simulink model "AR_Drone_Flight_Control"  (R2014a)
settings: configuration reference "AR_Drone_ConfigSet" (kept outside this file)
values from neighbouring files (symbols this model uses):
  Accelerometer_quick_calibration = [0.003485 0.008674 -0.9985]    [Calibration_Parameters.mat]
  Gyrometer_quick_calibration = [-10.63 2.778 -0.1868]    [Calibration_Parameters.mat]
undefined symbols (not defined in the file or in its folder): Accelerometer_360deg_calibration, Drone_StateModeType, Magnetometer_calibration, Navigation, Navigation_KF_Lib, sigbuilder_block
libraries: simulink x15, vrlib x7, aerolibtransform2 x5, AR_Drone_2_Library x4, dspnetwork x3, aerolibutil x2
(part 1 of 3)
settings Model: SimulationMode=external  ExtModeTrigDuration=48000  Creator=nraman  LastModifiedBy=Raphaël

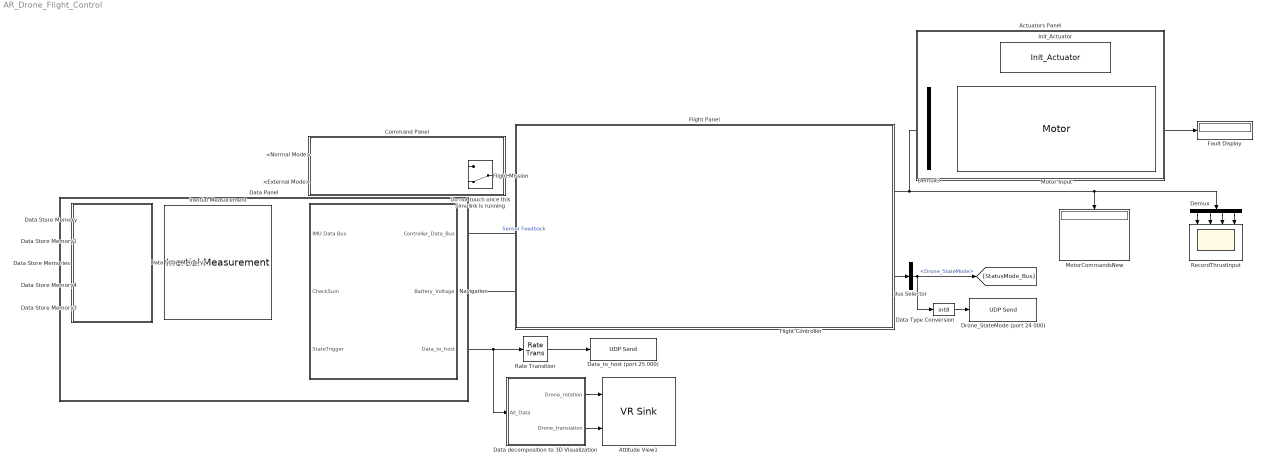
== system AR_Drone_Flight_Control ==
  <External Mode> : Subsystem
  <Normal Mode> : Subsystem
  Actuators Panel : Subsystem
  Attitude View1 : vrlib/VR Sink  InstantiateOnLoad=on  SampleTime=-1  ViewEnable=on  RemoteChange=off  RemoteView=off  FieldsWritten=Drone.rotation.4.1.1.double#Drone.translation.3.1.1.double  WorldFileName=myDrone3.wrl  AutoView=off  VideoDimensions=[]  AllowVariableSize=off
  Bus Selector : BusSelector  OutputSignals=Drone_StateMode
  Command Panel : Subsystem
  Data Panel : Subsystem
  Data Store Memory : DataStoreMemory  DataStoreName=Offset_Accel  ReadBeforeWriteMsg=warning  WriteAfterWriteMsg=warning  WriteAfterReadMsg=warning  InitialValue=[0 0 0]  OutDataTypeStr=double
  Data Store Memory1 : DataStoreMemory  DataStoreName=Offset_Gyro  ReadBeforeWriteMsg=warning  WriteAfterWriteMsg=warning  WriteAfterReadMsg=warning  InitialValue=[0 0 0]  OutDataTypeStr=double
  Data Store Memory2 : DataStoreMemory  DataStoreName=Input_ports  ReadBeforeWriteMsg=warning  WriteAfterWriteMsg=warning  WriteAfterReadMsg=warning  InitialValue=[0 0]  OutDataTypeStr=double
  Data Store Memory3 : DataStoreMemory  DataStoreName=Output_ports  ReadBeforeWriteMsg=warning  WriteAfterWriteMsg=warning  WriteAfterReadMsg=warning  InitialValue=[0 0]  OutDataTypeStr=double
  Data Store Memory4 : DataStoreMemory  DataStoreName=Flight_Mission_On_Off  ReadBeforeWriteMsg=warning  WriteAfterWriteMsg=warning  WriteAfterReadMsg=warning  InitialValue=false  OutDataTypeStr=boolean
  Data Store Memories : Subsystem
  Data Type Conversion : DataTypeConversion  OutDataTypeStr=int8
  Data decomposition to 3D Visualization : Subsystem
  Data_to_host (port 25 000) : dspnetwork/UDP Send  remoteURL=Host_IP_Adress  remotePort=25000  localURL='0.0.0.0'  localPortSource=Automatically determine  localPort=-1  sampletime=-1  blockPlatform=LINUX  separateLengthPort=0
  Demux : Demux
  Demux3 : Demux
  Do not touch once this Simulink is running : ManualSwitch  CurrentSetting=0
  Drone_StateMode (port 24 000) : dspnetwork/UDP Send  remoteURL=Host_IP_Adress  remotePort=24000  localURL='0.0.0.0'  localPortSource=Automatically determine  localPort=-1  sampletime=-1  blockPlatform=LINUX  separateLengthPort=0
  Fault Display : Display
  Flight Controller : Subsystem
  Flight Mission : Subsystem
  Flight Panel : Subsystem
  Inertial Measurement : AR_Drone_2_Library/Inertial Measurement  Ts=1/400
  Init_Actuator : AR_Drone_2_Library/Init_Actuator  ShowSpec=on
  Motor Input : AR_Drone_2_Library/Motor
  MotorCommandsNew : Display
  Navigation : Subsystem  AncestorBlock=Navigation_KF_Lib/Navigation
      mask DialogControl DescTextVar Prompt: Kalman Filter Navigation Implementation
  Rate Transition : RateTransition  OutPortSampleTime=2/400
  RecordThrustInput : Scope  NumInputPorts=4
      settings: TimeRange=44.32823813354787  YMin=20~20~-5~-5  YMax=85~90~5~5  SaveName=Control_Input
  wires:
  Motor Input/1 -> Fault Display/1
  Demux3/1 -> Motor Input/1
  Demux3/2 -> Motor Input/2
  Demux3/3 -> Motor Input/3
  Demux3/4 -> Motor Input/4
  Inertial Measurement/1 -> Navigation/1(IMU Data Bus)
  Inertial Measurement/2 -> Navigation/2(CheckSum)
  Flight Controller/2(ControlStatus_Bus) -> Bus Selector/1
  Demux/1 -> RecordThrustInput/1
  Demux/2 -> RecordThrustInput/2
  Navigation/1(Controller_Data_Bus) -> Flight Controller/2(Controller Feedback Data Bus)  "Sensor Feedback"
  Navigation/2(Battery_Voltage) -> Flight Controller/3(BatteryVoltage)
  [StatusMode_Bus] -> Navigation/3(StateTrigger)
  Navigation/3(Data_to_host) -> Rate Transition/1, Data decomposition to 3D Visualization/1(All_Data)
  Data decomposition to 3D Visualization/1(Drone_rotation) -> Attitude View1/1
  Data decomposition to 3D Visualization/2(Drone_translation) -> Attitude View1/2
  Flight Controller/1(MotorCommand) -> Demux3/1, MotorCommandsNew/1, Demux/1
  Demux/3 -> RecordThrustInput/3
  Demux/4 -> RecordThrustInput/4
  Bus Selector/1 -> [StatusMode_Bus], Data Type Conversion/1  "<Drone_StateMode>"
  Data Type Conversion/1 -> Drone_StateMode (port 24 000)/1
  Rate Transition/1 -> Data_to_host (port 25 000)/1
  Flight Mission/1(Command) -> Flight Controller/1(Command)
  <External Mode>/1("<External Mode> (on PC) : Switch") -> Do not touch once this Simulink is running/2
  Do not touch once this Simulink is running/1 -> Flight Mission/1(Start/Stop)
  <Normal Mode>/1("<Normal Mode> (Embedded) : UDP") -> Do not touch once this Simulink is running/1

== system AR_Drone_Flight_Control/<External Mode> ==
  " 1" : DataTypeConversion  OutDataTypeStr=int16
  Constant2 : Constant  Value=+1
  Constant3 : Constant  Value=-1
  Switch to change the current Drone State (it has to be down at the start) : ManualSwitch  CurrentSetting=0
  "<External Mode> (on PC) : Switch" : Outport
  wires:
  " 1"/1 -> "<External Mode> (on PC) : Switch"/1
  Switch to change the current Drone State (it has to be down at the start)/1 -> " 1"/1
  Constant2/1 -> Switch to change the current Drone State (it has to be down at the start)/1
  Constant3/1 -> Switch to change the current Drone State (it has to be down at the start)/2

== system AR_Drone_Flight_Control/<Normal Mode> ==
  " 1" : DataTypeConversion  OutDataTypeStr=int16
  Host Command (port 7 000) : dspnetwork/UDP Receive  localURL='0.0.0.0'  localPort=6000  remoteURL='0.0.0.0'  remotePort=-1  recvBufferSize=8192  dims=1  signalDatatype=double  isVarSize=off  showBlockingTime=on  blockingTime=0  sampletime=1/400  blockPlatform=LINUX
  Terminator2 : Terminator
  "<Normal Mode> (Embedded) : UDP" : Outport
  wires:
  Host Command (port 7 000)/2 -> Terminator2/1
  Host Command (port 7 000)/1 -> " 1"/1
  " 1"/1 -> "<Normal Mode> (Embedded) : UDP"/1

== system AR_Drone_Flight_Control/Actuators Panel ==

== system AR_Drone_Flight_Control/Command Panel ==

== system AR_Drone_Flight_Control/Data Panel ==

== system AR_Drone_Flight_Control/Data Store Memories ==

== system AR_Drone_Flight_Control/Data decomposition to 3D Visualization ==
  All_Data : Inport
  DCM (diagonal = 1 / else 0) : Display
      settings: Decimation=3
  Demux7 : Demux  Outputs=[13 9 3 3 3 3]
  Reshape : Reshape  OutputDimensionality=Customize  OutputDimensions=[3,3]
  SL3D Visualization1 : Subsystem
  Terminator2 : Terminator
  Terminator3 : Terminator
  Drone_rotation : Outport
  Drone_translation : Outport  Port=2
  wires:
  All_Data/1 -> Demux7/1
  Demux7/3 -> SL3D Visualization1/2(GravVector)
  Demux7/4 -> SL3D Visualization1/3(MagXY)
  Demux7/5 -> SL3D Visualization1/4(MagVector)
  Reshape/1 -> DCM (diagonal = 1 / else 0)/1, SL3D Visualization1/1(VisualizationInput)
  SL3D Visualization1/1(VRML_out) -> Drone_rotation/1
  SL3D Visualization1/2(VRML_pos) -> Drone_translation/1
  Demux7/2 -> Reshape/1
  Demux7/6 -> Terminator3/1
  Demux7/1 -> Terminator2/1

== system AR_Drone_Flight_Control/Flight Controller ==
  Command : Inport
  Controller Feedback Data Bus : Inport  Port=2
  BatteryVoltage : Inport  Port=3
  Bus Creator : BusCreator  Inputs=5
  Bus Selector : BusSelector  OutputSignals=UltraSound,EulerAngles,ProcessedGyro,AccelNorm
  Bus Selector1 : BusSelector  OutputSignals=Desired_Drone_StateMode,Auto-Calibration_ON_OFF,Altitude_ON_OFF,Desired_Roll_Pitch_Yaw
  Data Type Conversion1 : DataTypeConversion  OutDataTypeStr=int16
  Data Type Conversion3 : DataTypeConversion  OutDataTypeStr=int16
  Data Type Conversion4 : DataTypeConversion  OutDataTypeStr=int16
  Data Type Conversion5 : DataTypeConversion  OutDataTypeStr=boolean
  Drone_State-Mode Conversion : DataTypeConversion  OutDataTypeStr=Enum: Drone_StateModeType
  FilterBattVoltage : DiscreteTransferFcn  Numerator=[ 0.07226]  Denominator=[1 -0.9277]  SampleTime=1/400
  Nominal Thrust : Constant  Value=55  OutDataTypeStr=int16
  Selector : Selector  InputPortWidth=3  Indices=[3]
  Supervisory Flight Controller : Stateflow chart  TreatAsAtomicUnit=on
  MotorCommand : Outport
  ControlStatus_Bus : Outport  Port=2
  wires:
  Supervisory Flight Controller/1(MotorCmd) -> Bus Creator/1, MotorCommand/1
  Supervisory Flight Controller/2(" Drone_StateMode") -> Bus Creator/2
  Bus Selector/1 -> Supervisory Flight Controller/5(UltraSound_Feedback)  "<UltraSound>"
  Controller Feedback Data Bus/1 -> Bus Selector/1
  [Accel_data_for_offset] -> Supervisory Flight Controller/11(Accel_Measures_for_Offset)
  Supervisory Flight Controller/5(refHeight) -> Bus Creator/5
  [Gyro_data_for_offset] -> Supervisory Flight Controller/12(Gyro_Measures_for_Offset)
  BatteryVoltage/1 -> FilterBattVoltage/1
  FilterBattVoltage/1 -> Supervisory Flight Controller/10(Measured_Battery_Voltage)
  Selector/1 -> Supervisory Flight Controller/8(AccelVector_Input)
  Supervisory Flight Controller/3(" BatteryFault_Mode") -> Bus Creator/3
  Supervisory Flight Controller/4(" SafeOrientation_Mode") -> Bus Creator/4
  Bus Creator/1 -> ControlStatus_Bus/1  "StatusMode_Bus"
  Bus Selector/4 -> Selector/1  "<AccelNorm>"
  Bus Selector/2 -> Supervisory Flight Controller/6(Euler_Angles)  "<EulerAngles>"
  Bus Selector/3 -> Supervisory Flight Controller/7(Angular_Velocity)  "<ProcessedGyro>"
  Data Type Conversion1/1 -> Drone_State-Mode Conversion/1
  Drone_State-Mode Conversion/1 -> Supervisory Flight Controller/1(hostCmd)
  Data Type Conversion4/1 -> Supervisory Flight Controller/3(EnableAltitudeCtrl)
  Command/1 -> Bus Selector1/1
  Data Type Conversion5/1 -> Supervisory Flight Controller/2(Auto_Calibration)
  Nominal Thrust/1 -> Data Type Conversion3/1
  Data Type Conversion3/1 -> Supervisory Flight Controller/9(NominalThrust)
  Bus Selector1/1 -> Data Type Conversion1/1  "<Desired_Drone_StateMode>"
  Bus Selector1/4 -> Supervisory Flight Controller/4(Desired_Attitude_deg)  "<Desired_Roll_Pitch_Yaw>"
  Bus Selector1/3 -> Data Type Conversion4/1  "<Altitude_ON_OFF>"
  Bus Selector1/2 -> Data Type Conversion5/1  "<Auto-Calibration_ON_OFF>"

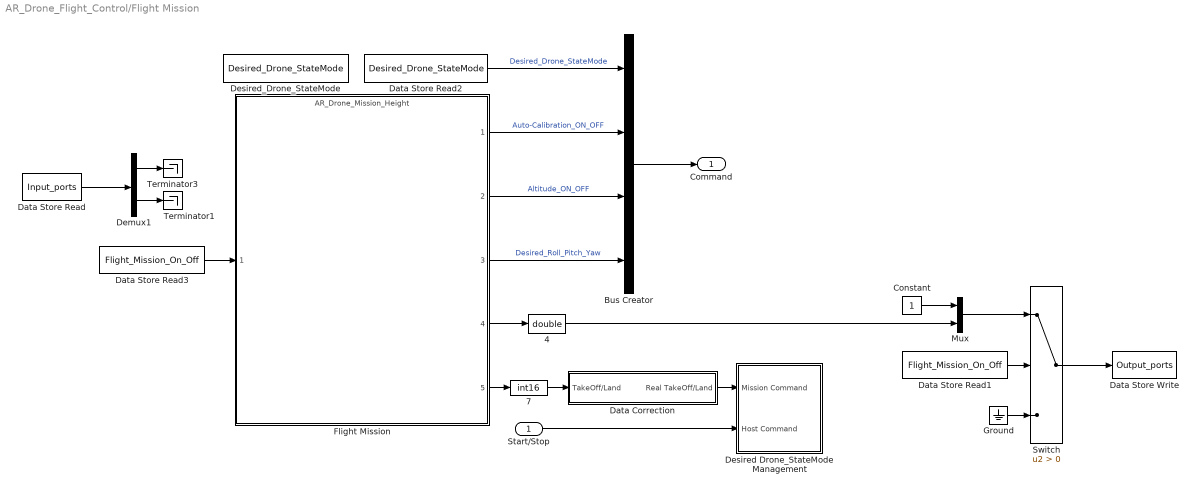
== system AR_Drone_Flight_Control/Flight Mission ==
  Start/Stop : Inport
  " 4" : DataTypeConversion  OutDataTypeStr=double
  " 7" : DataTypeConversion  OutDataTypeStr=int16
  Bus Creator : BusCreator
  Constant : Constant
  Data Correction : Subsystem
  Data Store Read : DataStoreRead  DataStoreName=Input_ports
  Data Store Read1 : DataStoreRead  DataStoreName=Flight_Mission_On_Off
  Data Store Read2 : DataStoreRead  DataStoreName=Desired_Drone_StateMode
  Data Store Read3 : DataStoreRead  DataStoreName=Flight_Mission_On_Off
  Data Store Write : DataStoreWrite  DataStoreName=Output_ports
  Demux1 : Demux  Outputs=2
  Desired Drone_StateMode Management : Subsystem
  Desired_Drone_StateMode : DataStoreMemory  DataStoreName=Desired_Drone_StateMode  ReadBeforeWriteMsg=warning  WriteAfterWriteMsg=warning  WriteAfterReadMsg=warning  InitialValue=Drone_StateModeType.Landing_Sequence  OutDataTypeStr=Enum: Drone_StateModeType
  Flight Mission : ModelReference  ModelNameDialog=AR_Drone_Mission_Height.slx  SimulationMode=Normal  ModelReferenceVersion=1.1120  CopyOfModelName=AR_Drone_Mission_Height.slx  DefaultDataLogging=on
  Ground : Ground
  Mux : Mux  Inputs=2
  Switch : Switch  Criteria=u2 > Threshold
  Terminator1 : Terminator
  Terminator3 : Terminator
  Command : Outport
  wires:
  Ground/1 -> Switch/3
  Flight Mission/5 -> " 7"/1
  Mux/1 -> Switch/1
  Constant/1 -> Mux/1
  Data Store Read3/1 -> Flight Mission/1
  Data Store Read/1 -> Demux1/1
  Demux1/2 -> Terminator1/1
  Switch/1 -> Data Store Write/1
  Flight Mission/1 -> Bus Creator/2  "Auto-Calibration_ON_OFF"
  Flight Mission/2 -> Bus Creator/3  "Altitude_ON_OFF"
  Flight Mission/3 -> Bus Creator/4  "Desired_Roll_Pitch_Yaw"
  Flight Mission/4 -> " 4"/1
  Start/Stop/1 -> Desired Drone_StateMode Management/2(Host Command)
  Data Store Read2/1 -> Bus Creator/1  "Desired_Drone_StateMode"
  " 4"/1 -> Mux/2
  " 7"/1 -> Data Correction/1(TakeOff/Land)
  Data Store Read1/1 -> Switch/2
  Data Correction/1(Real TakeOff/Land) -> Desired Drone_StateMode Management/1(Mission Command)
  Bus Creator/1 -> Command/1
  Demux1/1 -> Terminator3/1

== system AR_Drone_Flight_Control/Flight Panel ==

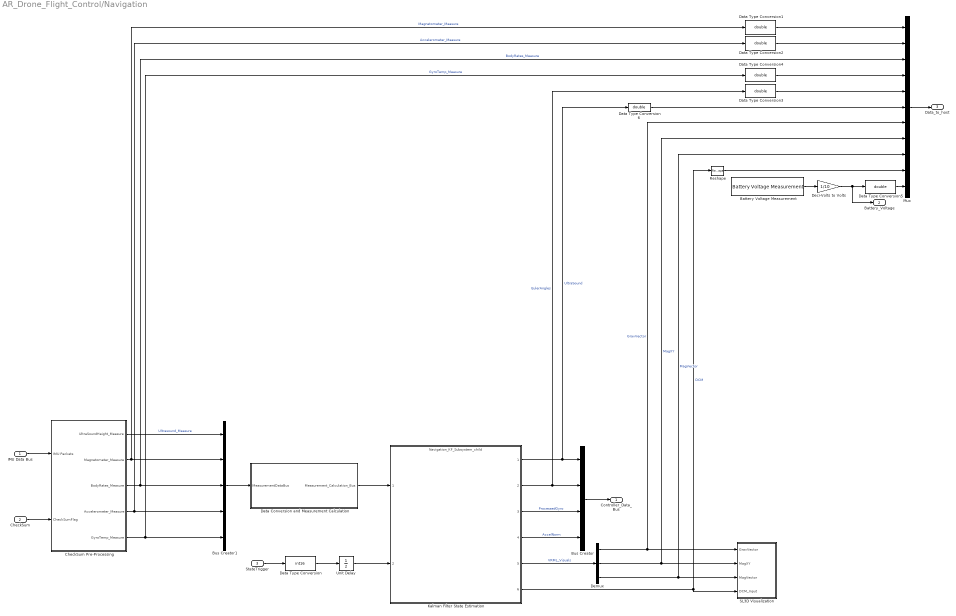
== system AR_Drone_Flight_Control/Navigation ==
  IMU Data Bus : Inport  OutDataTypeStr=Bus: IMU_Packets
  CheckSum : Inport  Port=2
  StateTrigger : Inport  Port=3  OutDataTypeStr=Enum: Drone_StateModeType
  Battery Voltage Measurement : AR_Drone_2_Library/Battery Voltage Measurement  SFunctionSpec=void BatteryMeasure_step(single y1[1])  SampleTime=1/400
  Bus Creator : BusCreator
  Bus Creator1 : BusCreator  Inputs=5
  CheckSum Pre-Processing : Subsystem  TreatAsAtomicUnit=on
      settings: RTWSystemCode=Inline
  Data Conversion and Measurement Calculation : Subsystem
  Data Type Conversion : DataTypeConversion  OutDataTypeStr=int16
  Data Type Conversion{1..6} (6 alike) : DataTypeConversion  OutDataTypeStr=double
  Deci-Volts to Volts : Gain  Gain=1/10
  Demux : Demux  Outputs=[3 3 3]
  Kalman Filter State Estimation : ModelReference  ModelNameDialog=Navigation_KF_Subsystem_child.slx  SimulationMode=Normal  ModelReferenceVersion=1.63  CopyOfModelName=Navigation_KF_Subsystem_child.slx  DefaultDataLogging=on
  Mux : Mux  Inputs=11
  Reshape : Reshape
  SL3D Visualization : Subsystem
  Unit Delay : UnitDelay  SampleTime=-1
  Controller_Data_Bus : Outport
  Battery_Voltage : Outport  Port=2
  Data_to_host : Outport  Port=3
  wires:
  Kalman Filter State Estimation/4 -> Bus Creator/4  "AccelNorm"
  Kalman Filter State Estimation/3 -> Bus Creator/3  "ProcessedGyro"
  StateTrigger/1 -> Data Type Conversion/1
  Bus Creator1/1 -> Data Conversion and Measurement Calculation/1(MeasurementDataBus)
  CheckSum Pre-Processing/5(GyroTemp_Measure) -> Data Type Conversion4/1, Bus Creator1/5  "GyroTemp_Measure"
  CheckSum Pre-Processing/4(Accelerometer_Measure) -> Data Type Conversion2/1, Bus Creator1/4  "Accelerometer_Measure"
  CheckSum Pre-Processing/3(BodyRates_Measure) -> Mux/3, Bus Creator1/3  "BodyRates_Measure"
  CheckSum Pre-Processing/2(Magnetometer_Measure) -> Data Type Conversion1/1, Bus Creator1/2  "Magnetometer_Measure"
  CheckSum Pre-Processing/1(UltraSoundHeight_Measure) -> Bus Creator1/1  "Ultrasound_Measure"
  CheckSum/1 -> CheckSum Pre-Processing/2(CheckSumFlag)
  IMU Data Bus/1 -> CheckSum Pre-Processing/1(IMU Packets)
  Unit Delay/1 -> Kalman Filter State Estimation/2
  Data Type Conversion/1 -> Unit Delay/1
  Kalman Filter State Estimation/1 -> Data Type Conversion6/1, Bus Creator/1  "UltraSound"
  Demux/1 -> Mux/7, SL3D Visualization/1(GravVector)  "GravVector"
  Demux/3 -> Mux/9, SL3D Visualization/3(MagVector)  "MagVector"
  Bus Creator/1 -> Controller_Data_Bus/1
  Kalman Filter State Estimation/2 -> Data Type Conversion3/1, Bus Creator/2  "EulerAngles"
  Kalman Filter State Estimation/5 -> Demux/1  "VRML_Visuals"
  Demux/2 -> Mux/8, SL3D Visualization/2(MagXY)  "MagXY"
  Data Conversion and Measurement Calculation/1(Measurement_Calculation_Bus) -> Kalman Filter State Estimation/1
  Kalman Filter State Estimation/6 -> SL3D Visualization/4(DCM_Input), Reshape/1  "DCM"
  Data Type Conversion4/1 -> Mux/4
  Data Type Conversion3/1 -> Mux/5
  Data Type Conversion2/1 -> Mux/2
  Data Type Conversion1/1 -> Mux/1
  Mux/1 -> Data_to_host/1
  Reshape/1 -> Mux/10
  Data Type Conversion6/1 -> Mux/6
  Battery Voltage Measurement/1 -> Deci-Volts to Volts/1
  Deci-Volts to Volts/1 -> Battery_Voltage/1, Data Type Conversion5/1
  Data Type Conversion5/1 -> Mux/11

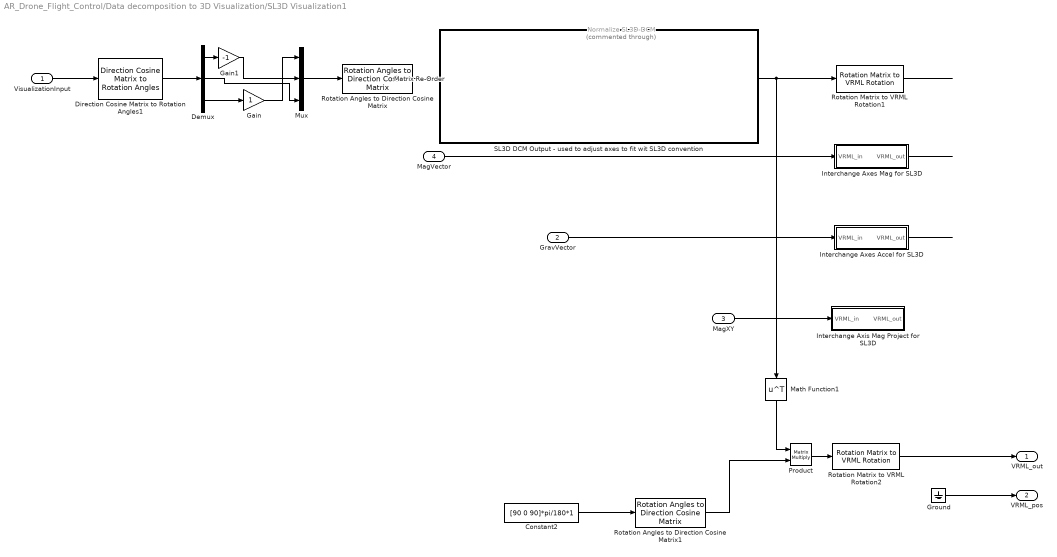
== system AR_Drone_Flight_Control/Data decomposition to 3D Visualization/SL3D Visualization1 ==
  VisualizationInput : Inport
  GravVector : Inport  Port=2
  MagXY : Inport  Port=3
  MagVector : Inport  Port=4
  Constant2 : Constant  Value=[90 0 90]*pi/180*1
  Demux : Demux  Outputs=3
  Direction Cosine Matrix to Rotation Angles1 : aerolibtransform2/Direction Cosine Matrix to Rotation Angles  rotationOrder=XYZ  lim=ZeroR3
      settings: AttributesFormatString=Rotation Order: %<rotationOrder>
  Gain : Gain  OutDataTypeStr=Inherit: Same as input
  Gain1 : Gain  Gain=-1  OutDataTypeStr=Inherit: Same as input
  Ground : Ground
  "Interchange Axes Accel for SL3D " : Subsystem
  "Interchange Axes Mag for SL3D " : Subsystem
  Interchange Axis Mag Project for SL3D : Subsystem
  Math Function1 : Math  Operator=transpose  SaturateOnIntegerOverflow=on
  Matrix Re-Order : MATLAB Function  TreatAsAtomicUnit=on
  Mux : Mux  Inputs=3
  Normalize SL3D-DCM : Subsystem  Commented=through  TreatAsAtomicUnit=on
  Product : Product  Multiplication=Matrix(*)
  Rotation Angles to Direction Cosine Matrix : aerolibtransform2/Rotation Angles to Direction Cosine Matrix  rotationOrder=XYZ
  Rotation Angles to Direction Cosine Matrix1 : aerolibtransform2/Rotation Angles to Direction Cosine Matrix  rotationOrder=XYZ
  Rotation Matrix to VRML Rotation1 : vrlib/Utilities/Rotation Matrix to VRML Rotation  maxzero=1e-12
  Rotation Matrix to VRML Rotation2 : vrlib/Utilities/Rotation Matrix to VRML Rotation  maxzero=1e-12
  SL3D DCM Output - used to adjust axes to fit wit SL3D convention : Subsystem
  VRML_out : Outport
  VRML_pos : Outport  Port=2
  wires:
  Rotation Matrix to VRML Rotation1/1 -> ?
  "Interchange Axes Accel for SL3D "/1(VRML_out) -> ?
  VisualizationInput/1 -> Direction Cosine Matrix to Rotation Angles1/1
  GravVector/1 -> "Interchange Axes Accel for SL3D "/1(VRML_in)
  Matrix Re-Order/1(M_out) -> Normalize SL3D-DCM/1(DCM)
  Direction Cosine Matrix to Rotation Angles1/1 -> Demux/1
  Demux/3 -> Gain/1
  Mux/1 -> Rotation Angles to Direction Cosine Matrix/1
  "Interchange Axes Mag for SL3D "/1(VRML_out) -> ?
  MagVector/1 -> "Interchange Axes Mag for SL3D "/1(VRML_in)
  Rotation Angles to Direction Cosine Matrix/1 -> Matrix Re-Order/1(M_in)
  MagXY/1 -> Interchange Axis Mag Project for SL3D/1(VRML_in)
  Rotation Matrix to VRML Rotation2/1 -> VRML_out/1
  Constant2/1 -> Rotation Angles to Direction Cosine Matrix1/1
  Rotation Angles to Direction Cosine Matrix1/1 -> Product/2
  Product/1 -> Rotation Matrix to VRML Rotation2/1
  Normalize SL3D-DCM/1(DCM_normalized) -> Math Function1/1, Rotation Matrix to VRML Rotation1/1
  Math Function1/1 -> Product/1
  Gain/1 -> Mux/1
  Demux/1 -> Gain1/1
  Demux/2 -> Mux/3
  Gain1/1 -> Mux/2
  Ground/1 -> VRML_pos/1

== system AR_Drone_Flight_Control/Flight Controller/Supervisory Flight Controller/Altitude_Control ==
  note: Thurst Table
      | _________________
      | At 100cm error  - 20% duty cycle - saturation : 10
      | 80 cm error - 16% duty cycle - saturation
      | 70 cm error - 14% duty cycle - saturation
      | 60 cm error - 12% duty cycle
  HeightFeedback : Inport  OutDataTypeStr=double  PortDimensions=2
  refHeight : Inport  Port=2  OutDataTypeStr=double  PortDimensions=1
  f : TriggerPort  TriggerType=function-call
      settings: CopyFcn=Stateflow.SLINSF.SimulinkMan.removeBlockPreDeleteFcn  PreDeleteFcn=Stateflow.SLINSF.SimulinkMan.unsafePredeleteFcn
  Control Effort : Scope
      settings: YMin=8.735  YMax=8.7875  SaveName=ScopeData3
  Data Type Conversion1 : DataTypeConversion  OutDataTypeStr=int16
  Demux : Demux  Outputs=2
  Discrete PID Controller _ WORKING1 : simulink/Continuous/PID Controller  Commented=on  Controller=PID  TimeDomain=Discrete-time  SampleTime=-1  IntegratorMethod=Forward Euler  FilterMethod=Forward Euler  Form=Parallel  P=0.387369235850492*0.7  I=0.018136*4  D=0.819231727791919*0.15  N=12.5907330811849  InitialConditionSource=internal  InitialConditionForIntegrator=0  InitialConditionForFilter=0  ExternalReset=none  LimitOutput=on  UpperSaturationLimit=20  LowerSaturationLimit=-20  LinearizeAsGain=off  AntiWindupMode=clamping  Kb=1  TrackingMode=off  Kt=1  PParamMin=[]  PParamMax=[]  IParamMin=[]  IParamMax=[]  DParamMin=[]  DParamMax=[]  NParamMin=[]  NParamMax=[]  KbParamMin=[]  KbParamMax=[]  KtParamMin=[]  KtParamMax=[]  POutMin=[]  POutMax=[]  IOutMin=[]  IOutMax=[]  DOutMin=[]  DOutMax=[]  NOutMin=[]  NOutMax=[]  KbOutMin=[]  KbOutMax=[]  KtOutMin=[]  KtOutMax=[]  IntegratorOutMin=[]  IntegratorOutMax=[]  FilterOutMin=[]  FilterOutMax=[]  SumOutMin=[]  SumOutMax=[]  SumI1OutMin=[]  SumI1OutMax=[]  SumI2OutMin=[]  SumI2OutMax=[]  SumI3OutMin=[]  SumI3OutMax=[]  SumDOutMin=[]  SumDOutMax=[]  SaturationOutMin=[]  SaturationOutMax=[]  IntegratorContinuousStateAttributes=''  IntegratorStateMustResolveToSignalObject=off  IntegratorRTWStateStorageClass=Auto  FilterContinuousStateAttributes=''  FilterStateMustResolveToSignalObject=off  FilterRTWStateStorageClass=Auto
  Display3 : Display
  Height Error : Scope  NumInputPorts=2
      settings: ShowLegends=on  YMin=-0.1075~-5  YMax=-0.08~5  SaveName=ScopeData13
  PID_Smooth : simulink/Continuous/PID Controller  Controller=PID  TimeDomain=Discrete-time  SampleTime=-1  IntegratorMethod=Forward Euler  FilterMethod=Forward Euler  Form=Parallel  P=0.387369235850492*0.9  I=0.018136*4  D=0.819231727791919*0.2  N=12.5907330811849  InitialConditionSource=internal  InitialConditionForIntegrator=0  InitialConditionForFilter=0  ExternalReset=none  LimitOutput=on  UpperSaturationLimit=20  LowerSaturationLimit=-20  LinearizeAsGain=off  AntiWindupMode=clamping  Kb=1  TrackingMode=off  Kt=1  PParamMin=[]  PParamMax=[]  IParamMin=[]  IParamMax=[]  DParamMin=[]  DParamMax=[]  NParamMin=[]  NParamMax=[]  KbParamMin=[]  KbParamMax=[]  KtParamMin=[]  KtParamMax=[]  POutMin=[]  POutMax=[]  IOutMin=[]  IOutMax=[]  DOutMin=[]  DOutMax=[]  NOutMin=[]  NOutMax=[]  KbOutMin=[]  KbOutMax=[]  KtOutMin=[]  KtOutMax=[]  IntegratorOutMin=[]  IntegratorOutMax=[]  FilterOutMin=[]  FilterOutMax=[]  SumOutMin=[]  SumOutMax=[]  SumI1OutMin=[]  SumI1OutMax=[]  SumI2OutMin=[]  SumI2OutMax=[]  SumI3OutMin=[]  SumI3OutMax=[]  SumDOutMin=[]  SumDOutMax=[]  SaturationOutMin=[]  SaturationOutMax=[]  IntegratorContinuousStateAttributes=''  IntegratorStateMustResolveToSignalObject=off  IntegratorRTWStateStorageClass=Auto  FilterContinuousStateAttributes=''  FilterStateMustResolveToSignalObject=off  FilterRTWStateStorageClass=Auto
  Re-Calibrate : Saturate  UpperLimit=200  LowerLimit=0  OutMin=0  OutMax=200
      settings: AttributesFormatString=|
      | Upper: %<UpperLimit>
      | Lower %<LowerLimit>
  Sum : Sum  Inputs=|-+
  deltaThrottle : Outport  OutDataTypeStr=int16
  wires:
  refHeight/1 -> Sum/2, Height Error/2, Display3/1  "Commanded"
  PID_Smooth/1 -> Control Effort/1, Data Type Conversion1/1
  Data Type Conversion1/1 -> deltaThrottle/1
  HeightFeedback/1 -> Demux/1
  Demux/1 -> Re-Calibrate/1
  Sum/1 -> PID_Smooth/1, Height Error/1  "Error"
  Re-Calibrate/1 -> Sum/1

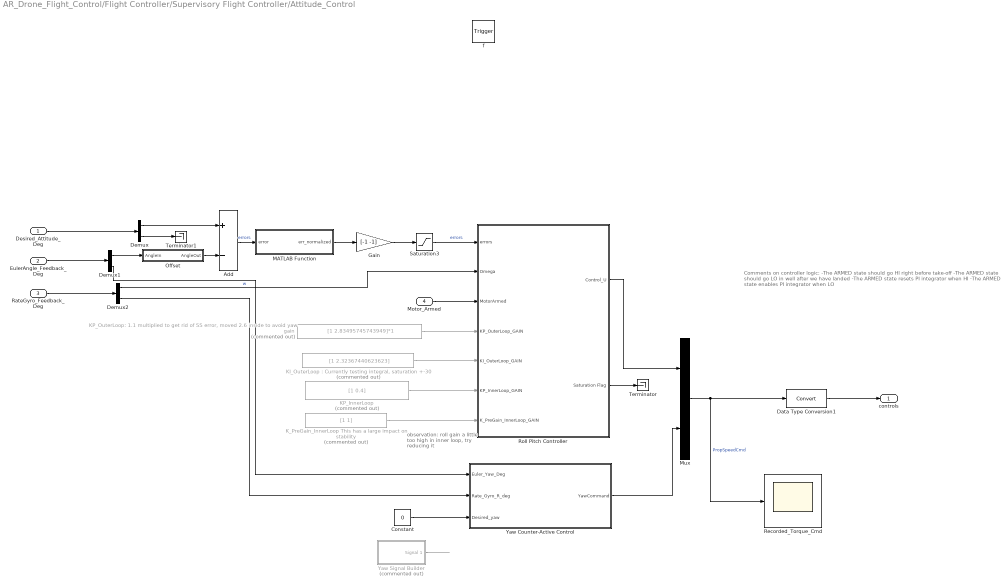
== system AR_Drone_Flight_Control/Flight Controller/Supervisory Flight Controller/Attitude_Control ==
  note: observation:
      | roll gain a little
      | too high in inner
      | loop, try reducing it
  note: Comments on controller logic:
      | -The ARMED state should go HI right before take-off
      | -The  ARMED state should go LO in well after we have landed
      | -The ARMED state resets PI integrator when HI
      | -The ARMED state enables PI integrator when LO
  Desired_Attitude_Deg : Inport  OutDataTypeStr=double  PortDimensions=3
  EulerAngle_Feedback_Deg : Inport  Port=2  OutDataTypeStr=double  PortDimensions=3
  RateGyro_Feedback_Deg : Inport  Port=3  OutDataTypeStr=double  PortDimensions=3
  Motor_Armed : Inport  Port=4  OutDataTypeStr=double  PortDimensions=1
  f : TriggerPort  TriggerType=function-call
      settings: CopyFcn=Stateflow.SLINSF.SimulinkMan.removeBlockPreDeleteFcn  PreDeleteFcn=Stateflow.SLINSF.SimulinkMan.unsafePredeleteFcn
  Add : Sum  Inputs=+-  AccumDataTypeStr=single  OutDataTypeStr=single
  Constant : Constant  Value=0
  Data Type Conversion1 : DataTypeConversion
  Demux : Demux  Outputs=[2 1]
  Demux1 : Demux  Outputs=[2 1]
  Demux2 : Demux  Outputs=[2 1]
  Gain : Gain  Gain=[-1 -1]
  "KI_OuterLoop : Currently testing integral, saturation +-30" : Constant  Commented=on  Value=[1 2.32367440623623]
  KP_InnerLoop : Constant  Commented=on  Value=[1 0.4]
  "KP_OuterLoop: 1.1 multiplied to get rid of SS error, moved 2.6 inside to avoid yaw gain" : Constant  Commented=on  Value=[1 2.83495745743949]*1
  K_PreGain_InnerLoop This has a large impact on stability : Constant  Commented=on  Value=[1 1]
  MATLAB Function : MATLAB Function  TreatAsAtomicUnit=on
  Mux : Mux  Inputs=2
  Offset : Subsystem
  Recorded_Torque_Cmd : Scope
      settings: TimeRange=30  YMin=-30  YMax=30  SaveName=Toqrue_Input
  Roll Pitch Controller : Subsystem  TreatAsAtomicUnit=on
  Saturation3 : Saturate  UpperLimit=[25 25]  LowerLimit=[-25 -25]  OutDataTypeStr=single
      settings: AttributesFormatString=%<LowerLimit> to %<UpperLimit>
  Terminator : Terminator
  Terminator1 : Terminator
  Yaw Counter-Active Control : Subsystem
  "Yaw Signal Builder " : Subsystem  Tag=STV Subsys  Commented=on  LoadFcn=sigbuilder_block('load');  StartFcn=sigbuilder_block('start');  StopFcn=sigbuilder_block('stop');  ClipboardFcn=sigbuilder_block('clipboard');  mask(Sigbuilder block){}
      mask help: Simulink:masks:SigbuilderBlock_MD
      mask init:
      | if ~strcmp(get_param(bdroot(gcbh),'SimulationStatus'),'stopped') tuvar = sigbuilder_block('maskInit'); end
      settings: CopyFcn=sigbuilder_block('copy');  DeleteFcn=sigbuilder_block('delete');  ModelCloseFcn=sigbuilder_block('modelClose');  PreSaveFcn=sigbuilder_block('preSave');  PauseFcn=sigbuilder_block('pause');  ContinueFcn=sigbuilder_block('continue');  NameChangeFcn=sigbuilder_block('namechange');  OpenFcn=sigbuilder_block('open',[437.25 118.5 550.5 394.5 ]);  CloseFcn=sigbuilder_block('close');
      mask Display: plot(0, 0, 100, 100,[2, 2, 32, 32, 2], [68, 8, 8, 68, 68],[32, 2], [38, 38], [32, 19, 2],[53, 60, 44], [32, 17, 17, 2],[16, 16, 31, 31]);txt = getActiveGroup(gcbh);text(2, 100, txt,'verticalAlignment', 'top');
  controls : Outport  OutDataTypeStr=int16  PortDimensions=3  InitialOutput=0
  wires:
  Add/1 -> MATLAB Function/1(error)  "errors"
  Demux1/1 -> Offset/1(AngleIn)
  Demux2/1 -> Roll Pitch Controller/2(Omega)  "w"
  KP_InnerLoop/1 -> Roll Pitch Controller/6(KP_InnerLoop_GAIN)
  "KP_OuterLoop: 1.1 multiplied to get rid of SS error, moved 2.6 inside to avoid yaw gain"/1 -> Roll Pitch Controller/4(KP_OuterLoop_GAIN)
  K_PreGain_InnerLoop This has a large impact on stability/1 -> Roll Pitch Controller/7(K_PreGain_InnerLoop_GAIN)
  "KI_OuterLoop : Currently testing integral, saturation +-30"/1 -> Roll Pitch Controller/5(KI_OuterLoop_GAIN)
  Saturation3/1 -> Roll Pitch Controller/1(errors)  "errors"
  MATLAB Function/1(err_normalized) -> Gain/1
  Gain/1 -> Saturation3/1
  Roll Pitch Controller/2(Saturation Flag) -> Terminator/1
  Demux/1 -> Add/1
  Roll Pitch Controller/1(Control_U) -> Mux/1
  Demux/2 -> Terminator1/1
  Offset/1(AngleOut) -> Add/2
  Demux2/2 -> Yaw Counter-Active Control/2(Rate_Gyro_R_deg)
  Yaw Counter-Active Control/1(YawCommand) -> Mux/2
  Desired_Attitude_Deg/1 -> Demux/1
  EulerAngle_Feedback_Deg/1 -> Demux1/1
  RateGyro_Feedback_Deg/1 -> Demux2/1
  Motor_Armed/1 -> Roll Pitch Controller/3(MotorArmed)
  Demux1/2 -> Yaw Counter-Active Control/1(Euler_Yaw_Deg)
  Data Type Conversion1/1 -> controls/1
  Mux/1 -> Data Type Conversion1/1, Recorded_Torque_Cmd/1  "PropSpeedCmd"
  "Yaw Signal Builder "/1(Signal 1) -> ?
  Constant/1 -> Yaw Counter-Active Control/3("Desired_yaw ")

== system AR_Drone_Flight_Control/Flight Controller/Supervisory Flight Controller/Drone_State.WaitForHost.checkConvergence ==
  Euler_Angles : Inport  OutDataTypeStr=double  PortDimensions=3
  f : TriggerPort  TriggerType=function-call
      settings: CopyFcn=Stateflow.SLINSF.SimulinkMan.removeBlockPreDeleteFcn  PreDeleteFcn=Stateflow.SLINSF.SimulinkMan.unsafePredeleteFcn
  Compare To Constant : simulink/Logic and Bit Operations/Compare To Constant  relop=<  const=0.00001  OutDataTypeStr=boolean
  Delay : Delay  DelayLength=1  InitialCondition=inf
  Demux : Demux  Outputs=3
  Display : Display
  Logical Operator : Logic  Inputs=3  AllPortsSameDT=off  OutDataTypeStr=boolean
  Sum : Sum  Inputs=|+-
  dt : Gain  Gain=1/400
  converge : Outport
  wires:
  Euler_Angles/1 -> Sum/2, Delay/1
  Delay/1 -> Sum/1
  Sum/1 -> dt/1
  dt/1 -> Compare To Constant/1
  Compare To Constant/1 -> Display/1, Demux/1
  Logical Operator/1 -> converge/1
  Demux/1 -> Logical Operator/1
  Demux/2 -> Logical Operator/2
  Demux/3 -> Logical Operator/3

== system AR_Drone_Flight_Control/Flight Controller/Supervisory Flight Controller/Drone_State.WaitForHost.checkMove ==
  Euler_Angles : Inport  OutDataTypeStr=double  PortDimensions=3
  f : TriggerPort  TriggerType=function-call
      settings: CopyFcn=Stateflow.SLINSF.SimulinkMan.removeBlockPreDeleteFcn  PreDeleteFcn=Stateflow.SLINSF.SimulinkMan.unsafePredeleteFcn
  Abs : Abs
  Compare To Constant : simulink/Logic and Bit Operations/Compare To Constant  relop=<  const=50  OutDataTypeStr=boolean
  Delay : Delay  DelayLength=40  InitialCondition=inf
  Demux : Demux  Outputs=3
  Display : Display
  Logical Operator : Logic  Inputs=3  AllPortsSameDT=off  OutDataTypeStr=boolean
  Logical Operator1 : Logic  Operator=NOT  AllPortsSameDT=off  OutDataTypeStr=boolean
  Scope1 : Scope
      settings: SaveName=Difference
  Scope3 : Scope
      settings: SaveName=Move
  Sum : Sum  Inputs=|+-
  move : Outport
  wires:
  Euler_Angles/1 -> Sum/2, Delay/1
  Delay/1 -> Sum/1
  Sum/1 -> Abs/1
  Compare To Constant/1 -> Display/1, Demux/1
  Logical Operator/1 -> Logical Operator1/1
  Demux/1 -> Logical Operator/1
  Demux/2 -> Logical Operator/2
  Demux/3 -> Logical Operator/3
  Logical Operator1/1 -> Scope3/1, move/1
  Abs/1 -> Scope1/1, Compare To Constant/1

== system AR_Drone_Flight_Control/Flight Controller/Supervisory Flight Controller/Motor_Mixing ==
  note: AR Drone:
      |
      |   1x         2y
      |      drone
      |   4y         3x
      |
      |  1 = constrain(throttle + 0.5*roll - 0.5*pitch - yaw , minThrottle, 30);
      |  2 = constrain(throttle - 0.5*roll - 0.5*pitch + yaw, minThrottle, 30);
      |  3 = constrain(throttle - 0.5*roll + 0.5*pitch - yaw, minThrottle, 30);
      |  4 = constrain(throttle + 0.5*roll + 0.5*pitch + yaw, minThrottle, 30);
  throttle : Inport  OutDataTypeStr=int16  PortDimensions=1
  RPYCmd : Inport  Port=2  OutDataTypeStr=int16  PortDimensions=3
  LandingPhase : Inport  Port=3  OutDataTypeStr=double  PortDimensions=1
  Motor_Armed : Inport  Port=4  OutDataTypeStr=double  PortDimensions=1
  f : TriggerPort  TriggerType=function-call
      settings: CopyFcn=Stateflow.SLINSF.SimulinkMan.removeBlockPreDeleteFcn  PreDeleteFcn=Stateflow.SLINSF.SimulinkMan.unsafePredeleteFcn
  Constant : Constant  Value=100  OutDataTypeStr=int16  SampleTime=-1
  Constant1 : Constant  Value=[0 0 0 0]  OutDataTypeStr=int16
  Constant2 : Constant  Value=[55 55 55 55]*0.4
  Data Type Conversion : DataTypeConversion  OutDataTypeStr=double
  Gain : Gain  Gain=[1 1 -1 -1; 1 -1 -1 1; 1 -1 1 -1; 1 1 1 1]  Multiplication=Matrix(K*u)  ParamDataTypeStr=int16  OutDataTypeStr=int16
  Logical Operator1 : Logic  Operator=NOT  AllPortsSameDT=off  OutDataTypeStr=boolean
  Mux1 : Mux  Inputs=2
  RampDownInSpeed1 : MATLAB Function  TreatAsAtomicUnit=on
  Saturation Dynamic : simulink/Discontinuities/Saturation Dynamic  OutMin=[]  OutMax=[]  OutDataTypeStr=Inherit: Same as second input  OutDataType=fixdt(1, 16)  OutScaling=2^-10  DoSatur=off
  Switch : Switch  Criteria=u2 > Threshold
  Switch1 : Switch  Criteria=u2 > Threshold
  minThrottle : Constant  Value=10  OutDataTypeStr=int16
  MotorCommands : Outport  InitialOutput=0
  wires:
  RPYCmd/1 -> Mux1/2
  minThrottle/1 -> Saturation Dynamic/3
  Constant/1 -> Saturation Dynamic/1
  Mux1/1 -> Gain/1
  Gain/1 -> Saturation Dynamic/2
  throttle/1 -> Mux1/1
  Data Type Conversion/1 -> RampDownInSpeed1/1(Cmd)
  RampDownInSpeed1/1(motorCmd) -> Switch/3
  Constant2/1 -> Data Type Conversion/1
  LandingPhase/1 -> RampDownInSpeed1/2(stopCmd), Logical Operator1/1  "if 1==Land, if 0 == dont land"
  Switch/1 -> MotorCommands/1
  Logical Operator1/1 -> Switch/2
  Saturation Dynamic/1 -> Switch1/1
  Motor_Armed/1 -> Switch1/2
  Constant1/1 -> Switch1/3
  Switch1/1 -> Switch/1

== system AR_Drone_Flight_Control/Flight Mission/Data Correction ==
  note: This Subsystem tests if a StateMode change must be done :
      | - If the Desired StateMode is Controlled_Flight and the Mission tells to land (-1), a change must be done
      | - If the Desired StateMode is Landing_Sequence and the Mission tells to take off (+1), a change must be done
      | - Else, no change must be done
  TakeOff/Land : Inport
  Change Desired Drone_StateMode : Constant  OutDataTypeStr=int16
  Constant1 : Constant  Value=-1
  Constant2 : Constant  Value=+1
  Data Store Read1 : DataStoreRead  DataStoreName=Desired_Drone_StateMode
  Data Store Read3 : DataStoreRead  DataStoreName=Desired_Drone_StateMode
  Don't change Desired Drone_StateMode : Constant  Value=0  OutDataTypeStr=int16
  Enumerated Constant : simulink/Sources/Enumerated Constant  OutDataTypeStr=Enum: Drone_StateModeType  Value=Drone_StateModeType.Controlled_Flight  SampleTime=inf
      settings: AttributesFormatString=%<Value>
  Enumerated Constant1 : simulink/Sources/Enumerated Constant  OutDataTypeStr=Enum: Drone_StateModeType  Value=Drone_StateModeType.Landing_Sequence  SampleTime=inf
      settings: AttributesFormatString=%<Value>
  Logical Operator : Logic  Operator=OR  AllPortsSameDT=off  OutDataTypeStr=boolean
  Logical Operator2 : Logic  AllPortsSameDT=off  OutDataTypeStr=boolean
  Logical Operator3 : Logic  AllPortsSameDT=off  OutDataTypeStr=boolean
  Switch1 : Switch  Criteria=u2 > Threshold
  Tests if Desired_Drone_StateMode is Contrelled_Flight : RelationalOperator  Operator===  OutDataTypeStr=boolean
  Tests if Desired_Drone_StateMode is Landing_Sequence : RelationalOperator  Operator===  OutDataTypeStr=boolean
  Tests if data equals +1 : RelationalOperator  Operator===  OutDataTypeStr=boolean
  Tests if data equals -1 : RelationalOperator  Operator===  OutDataTypeStr=boolean
  Real TakeOff/Land : Outport
  wires:
  TakeOff/Land/1 -> Tests if data equals -1/2, Tests if data equals +1/1
  Constant1/1 -> Tests if data equals -1/1
  Constant2/1 -> Tests if data equals +1/2
  Logical Operator/1 -> Switch1/2
  Switch1/1 -> Real TakeOff/Land/1
  Tests if data equals -1/1 -> Logical Operator3/2
  Tests if data equals +1/1 -> Logical Operator2/1
  Data Store Read1/1 -> Tests if Desired_Drone_StateMode is Contrelled_Flight/2
  Enumerated Constant/1 -> Tests if Desired_Drone_StateMode is Contrelled_Flight/1
  Data Store Read3/1 -> Tests if Desired_Drone_StateMode is Landing_Sequence/2
  Enumerated Constant1/1 -> Tests if Desired_Drone_StateMode is Landing_Sequence/1
  Tests if Desired_Drone_StateMode is Contrelled_Flight/1 -> Logical Operator3/1
  Tests if Desired_Drone_StateMode is Landing_Sequence/1 -> Logical Operator2/2
  Logical Operator3/1 -> Logical Operator/1
  Logical Operator2/1 -> Logical Operator/2
  Change Desired Drone_StateMode/1 -> Switch1/1
  Don't change Desired Drone_StateMode/1 -> Switch1/3

== system AR_Drone_Flight_Control/Flight Mission/Desired Drone_StateMode Management ==
  note: This Subsystem modifies the value of "Desired_Drone_StateMode" if the input data changes
      | (from -1 to +1 or from +1 to -1). "Derired_Drone_StateMode" should have 2 possible values :
      | "LandingSequence" (=3) or "Controlled Flight" (=2), so the initial condition is 3 ("LandingSequence")
      |
      | This integrates also the changing command from the flight mission, but the host command has a higher priority
  Mission Command : Inport
  Host Command : Inport  Port=2
  " 2" : DataTypeConversion  OutDataTypeStr=boolean
  " 3" : DataTypeConversion  OutDataTypeStr=int16
  " 4" : DataTypeConversion  OutDataTypeStr=int16
  " 5" : DataTypeConversion  OutDataTypeStr=int16
  Abs : Abs
  Constant : Constant  Value=2  OutDataTypeStr=int16
  Data Correction : Subsystem
  Data Store Read3 : DataStoreRead  DataStoreName=Desired_Drone_StateMode
  Data Store Write1 : DataStoreWrite  DataStoreName=Desired_Drone_StateMode
  Drone_State-Mode Conversion : DataTypeConversion  OutDataTypeStr=Enum: Drone_StateModeType
  Host Command > Mission Command : Gain  Gain=2
  Math Function : Math  Operator=mod  SaturateOnIntegerOverflow=on
  Memory : Memory  X0=-1
  Sum : Sum  Inputs=|+-
  Sum1 : Sum  Inputs=++|
  Sum2 : Sum  Inputs=++|
  Sum4 : Sum  Inputs=++|
  wires:
  Memory/1 -> Sum/2
  Host Command/1 -> Data Correction/1(Start/Stop)
  Data Correction/1(Real Start/Stop) -> Memory/1, Sum/1
  Data Store Read3/1 -> " 5"/1
  Sum2/1 -> Math Function/1
  Math Function/1 -> Sum1/2
  Drone_State-Mode Conversion/1 -> Data Store Write1/1
  " 5"/1 -> Sum2/1
  Abs/1 -> " 4"/1
  Constant/1 -> Sum1/1, Math Function/2
  Sum1/1 -> Drone_State-Mode Conversion/1
  " 2"/1 -> " 3"/1
  " 3"/1 -> Sum2/2
  " 4"/1 -> " 2"/1
  Sum/1 -> Host Command > Mission Command/1
  Sum4/1 -> Abs/1
  Host Command > Mission Command/1 -> Sum4/2
  Mission Command/1 -> Sum4/1

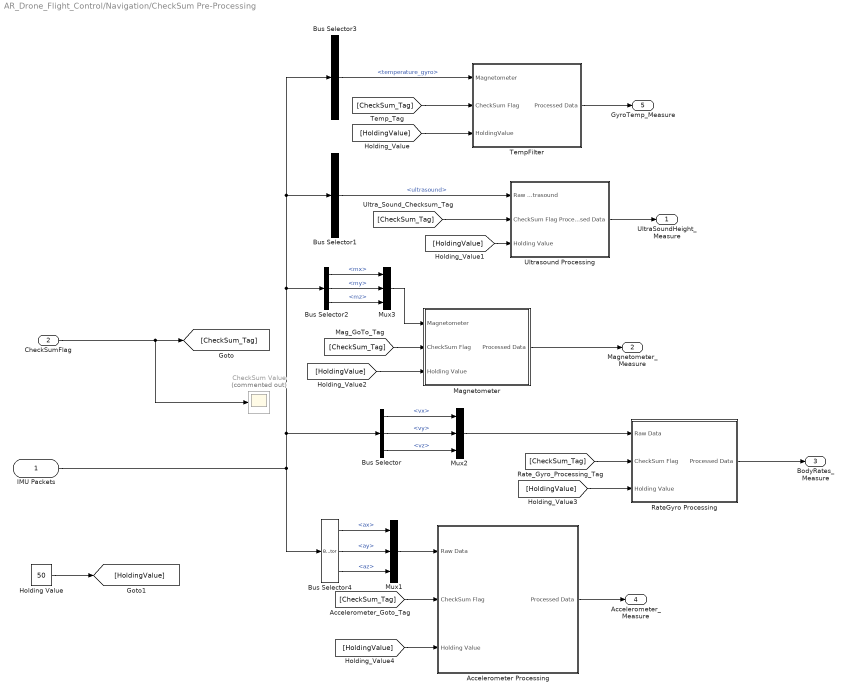
== system AR_Drone_Flight_Control/Navigation/CheckSum Pre-Processing ==
  IMU Packets : Inport
  CheckSumFlag : Inport  Port=2
  Accelerometer Processing : Subsystem
  Bus Selector : BusSelector  OutputSignals=vx,vy,vz
  Bus Selector1 : BusSelector  OutputSignals=ultrasound
  Bus Selector2 : BusSelector  OutputSignals=mx,my,mz
  Bus Selector3 : BusSelector  OutputSignals=temperature_gyro
  Bus Selector4 : BusSelector  OutputSignals=ax,ay,az
  CheckSum Value : Scope  Commented=on
      settings: YMin=0  YMax=2500  SaveName=CheckSum
  Holding Value : Constant  Value=50
  Magnetometer : Subsystem
  Mux1 : Mux  Inputs=3
  Mux2 : Mux  Inputs=3
  Mux3 : Mux  Inputs=3
  RateGyro Processing : Subsystem
  TempFilter : Subsystem
  Ultrasound Processing : Subsystem
  UltraSoundHeight_Measure : Outport
  Magnetometer_Measure : Outport  Port=2
  BodyRates_Measure : Outport  Port=3
  Accelerometer_Measure : Outport  Port=4
  GyroTemp_Measure : Outport  Port=5
  wires:
  Mux3/1 -> Magnetometer/1(Magnetometer)
  Holding Value/1 -> [HoldingValue]
  [HoldingValue] -> Accelerometer Processing/3(Holding Value)
  [HoldingValue] -> RateGyro Processing/3(Holding Value)
  [HoldingValue] -> Magnetometer/3(Holding Value)
  [HoldingValue] -> Ultrasound Processing/3(Holding Value)
  [HoldingValue] -> TempFilter/3(HoldingValue)
  [CheckSum_Tag] -> TempFilter/2(CheckSum Flag)
  TempFilter/1(Processed Data) -> GyroTemp_Measure/1
  Bus Selector3/1 -> TempFilter/1(Magnetometer)  "<temperature_gyro>"
  Bus Selector/3 -> Mux2/3  "<vz>"
  Bus Selector/2 -> Mux2/2  "<vy>"
  Bus Selector/1 -> Mux2/1  "<vx>"
  Ultrasound Processing/1(Processed Data) -> UltraSoundHeight_Measure/1
  [CheckSum_Tag] -> Accelerometer Processing/2(CheckSum Flag)
  Magnetometer/1(Processed Data) -> Magnetometer_Measure/1
  [CheckSum_Tag] -> Magnetometer/2(CheckSum Flag)
  Bus Selector2/3 -> Mux3/3  "<mz>"
  Bus Selector2/2 -> Mux3/2  "<my>"
  Bus Selector2/1 -> Mux3/1  "<mx>"
  RateGyro Processing/1(Processed Data) -> BodyRates_Measure/1
  [CheckSum_Tag] -> RateGyro Processing/2(CheckSum Flag)
  Mux2/1 -> RateGyro Processing/1(Raw Data)
  Accelerometer Processing/1(Processed Data) -> Accelerometer_Measure/1
  [CheckSum_Tag] -> Ultrasound Processing/2(CheckSum Flag)
  Mux1/1 -> Accelerometer Processing/1(Raw Data)
  Bus Selector4/3 -> Mux1/3  "<az>"
  Bus Selector4/2 -> Mux1/2  "<ay>"
  Bus Selector4/1 -> Mux1/1  "<ax>"
  IMU Packets/1 -> Bus Selector4/1, Bus Selector2/1, Bus Selector1/1, Bus Selector3/1, Bus Selector/1
  CheckSumFlag/1 -> CheckSum Value/1, [CheckSum_Tag]
  Bus Selector1/1 -> Ultrasound Processing/1(Raw Ultrasound)  "<ultrasound>"

== system AR_Drone_Flight_Control/Navigation/Data Conversion and Measurement Calculation ==
  MeasurementDataBus : Inport
  Bus Creator1 : BusCreator
  Bus Selector : BusSelector  OutputSignals=Ultrasound_Measure,Accelerometer_Measure,BodyRates_Measure,Magnetometer_Measure
  Calculate Gravity Vector : Subsystem
  Calibration_Scale_and_Offset : Subsystem
  Data Store Read1 : DataStoreRead  DataStoreName=Offset_Gyro
  Data Store Read2 : DataStoreRead  DataStoreName=Offset_Accel
  Remove Offset : Subsystem
  Signal Specification : SignalSpecification
  Measurement_Calculation_Bus : Outport
  wires:
  MeasurementDataBus/1 -> Bus Selector/1
  Bus Selector/4 -> Calibration_Scale_and_Offset/1(RawMag)  "<Magnetometer_Measure>"
  Data Store Read2/1 -> Calculate Gravity Vector/2(Accel_Offset)
  Data Store Read1/1 -> Remove Offset/2(Gyro Offset)
  Bus Selector/3 -> Remove Offset/1(Raw Gyro Values)  "<BodyRates_Measure>"
  Bus Selector/1 -> Signal Specification/1  "<Ultrasound_Measure>"
  Calibration_Scale_and_Offset/1(Normalized  Magnetometer) -> Bus Creator1/4  "Magnetometer_Calculation"
  Remove Offset/1(Gyro Offset Remove) -> Bus Creator1/3  "Gyro_Calculation"
  Signal Specification/1 -> Bus Creator1/1  "UltraSound_Calculation"
  Calculate Gravity Vector/1(Accel_Norm) -> Bus Creator1/2  "AccelNorm_Calculation"
  Bus Creator1/1 -> Measurement_Calculation_Bus/1
  Bus Selector/2 -> Calculate Gravity Vector/1(Accel)  "<Accelerometer_Measure>"

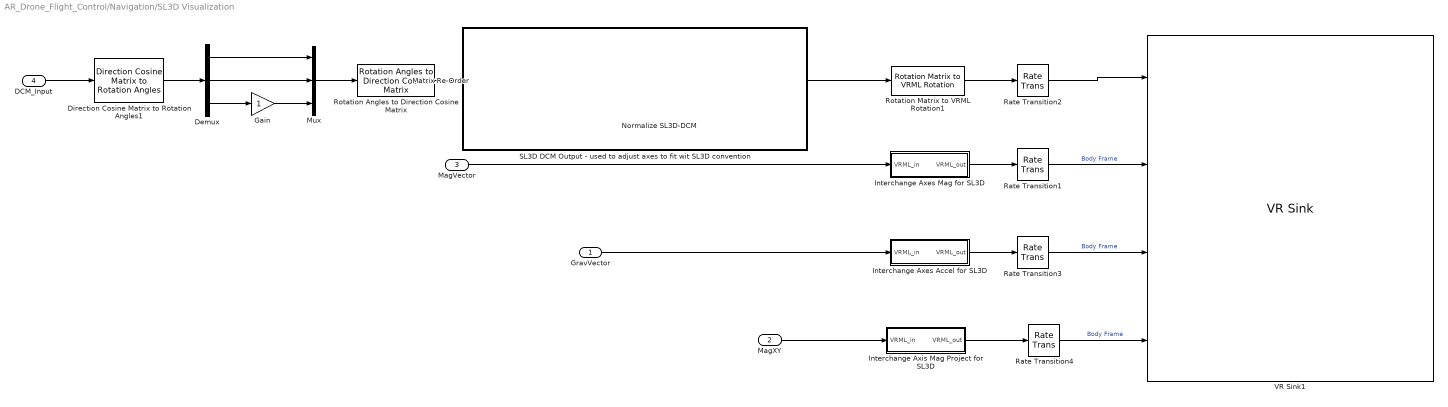
== system AR_Drone_Flight_Control/Navigation/SL3D Visualization ==
  GravVector : Inport
  MagXY : Inport  Port=2
  MagVector : Inport  Port=3
  DCM_Input : Inport  Port=4
  Demux : Demux  Outputs=3
  Direction Cosine Matrix to Rotation Angles1 : aerolibtransform2/Direction Cosine Matrix to Rotation Angles  rotationOrder=XYZ  lim=ZeroR3
      settings: AttributesFormatString=Rotation Order: %<rotationOrder>
  Gain : Gain  OutDataTypeStr=Inherit: Same as input
  "Interchange Axes Accel for SL3D " : Subsystem
  "Interchange Axes Mag for SL3D " : Subsystem
  Interchange Axis Mag Project for SL3D : Subsystem
  Matrix Re-Order : MATLAB Function  TreatAsAtomicUnit=on
  Mux : Mux  Inputs=3
  Normalize SL3D-DCM : Subsystem  TreatAsAtomicUnit=on
  Rate Transition{1..4} (4 alike) : RateTransition
  Rotation Angles to Direction Cosine Matrix : aerolibtransform2/Rotation Angles to Direction Cosine Matrix  rotationOrder=XYZ
  Rotation Matrix to VRML Rotation1 : vrlib/Utilities/Rotation Matrix to VRML Rotation  maxzero=1e-12
  SL3D DCM Output - used to adjust axes to fit wit SL3D convention : Subsystem
  VR Sink1 : vrlib/VR Sink  InstantiateOnLoad=on  SampleTime=0.02  ViewEnable=on  RemoteChange=off  RemoteView=off  FieldsWritten=Plane.rotation.4.1.1.double#mag_point.translation.3.1.1.double#grav_point.translation.3.1.1.double#mag_projection_point.translation.3.1.1.double  WorldFileName=vrml8_grav_2.WRL  AutoView=off  VideoDimensions=[]  AllowVariableSize=off
  wires:
  MagXY/1 -> Interchange Axis Mag Project for SL3D/1(VRML_in)
  Rate Transition2/1 -> VR Sink1/1
  Rate Transition1/1 -> VR Sink1/2  "Body Frame"
  Rate Transition3/1 -> VR Sink1/3  "Body Frame"
  Rate Transition4/1 -> VR Sink1/4  "Body Frame"
  Interchange Axis Mag Project for SL3D/1(VRML_out) -> Rate Transition4/1
  Rotation Angles to Direction Cosine Matrix/1 -> Matrix Re-Order/1(M_in)
  MagVector/1 -> "Interchange Axes Mag for SL3D "/1(VRML_in)
  "Interchange Axes Mag for SL3D "/1(VRML_out) -> Rate Transition1/1
  Mux/1 -> Rotation Angles to Direction Cosine Matrix/1
  Gain/1 -> Mux/3
  Demux/3 -> Gain/1
  Demux/2 -> Mux/2
  Demux/1 -> Mux/1
  Direction Cosine Matrix to Rotation Angles1/1 -> Demux/1
  Normalize SL3D-DCM/1(DCM_normalized) -> Rotation Matrix to VRML Rotation1/1
  Matrix Re-Order/1(M_out) -> Normalize SL3D-DCM/1(DCM)
  GravVector/1 -> "Interchange Axes Accel for SL3D "/1(VRML_in)
  DCM_Input/1 -> Direction Cosine Matrix to Rotation Angles1/1
  "Interchange Axes Accel for SL3D "/1(VRML_out) -> Rate Transition3/1
  Rotation Matrix to VRML Rotation1/1 -> Rate Transition2/1

== system AR_Drone_Flight_Control/Data decomposition to 3D Visualization/SL3D Visualization1/Interchange Axes Accel for SL3D  ==
  VRML_in : Inport
  Demux1 : Demux  Outputs=3
  Gain1 : Gain  Gain=3
  Gain2 : Gain
  Gain3 : Gain
  Mux2 : Mux  Inputs=3
  VRML_out : Outport
  wires:
  Gain1/1 -> Demux1/1
  Demux1/1 -> Gain3/1
  Demux1/3 -> Mux2/2
  Gain2/1 -> Mux2/1
  Gain3/1 -> Mux2/3
  Mux2/1 -> VRML_out/1
  Demux1/2 -> Gain2/1
  VRML_in/1 -> Gain1/1

== system AR_Drone_Flight_Control/Data decomposition to 3D Visualization/SL3D Visualization1/Interchange Axes Mag for SL3D  ==
  VRML_in : Inport
  Home Drone : Subsystem
  Subsystem : Subsystem  Commented=on
  Work Drone : Subsystem
  Work Drone - supposed work drone .. not really : Subsystem
  VRML_out : Outport
  wires:
  VRML_in/1 -> Work Drone/1(In1), Home Drone/1(In1)
  Work Drone/1(Out1) -> VRML_out/1

== system AR_Drone_Flight_Control/Data decomposition to 3D Visualization/SL3D Visualization1/Interchange Axis Mag Project for SL3D ==
  VRML_in : Inport
  Demux1 : Demux  Outputs=3
  Gain2 : Gain
  Gain3 : Gain
  Mux2 : Mux  Inputs=3
  VRML_out : Outport
  wires:
  VRML_in/1 -> Demux1/1
  Demux1/1 -> Gain3/1
  Demux1/3 -> Mux2/2
  Gain2/1 -> Mux2/1
  Gain3/1 -> Mux2/3
  Mux2/1 -> VRML_out/1
  Demux1/2 -> Gain2/1

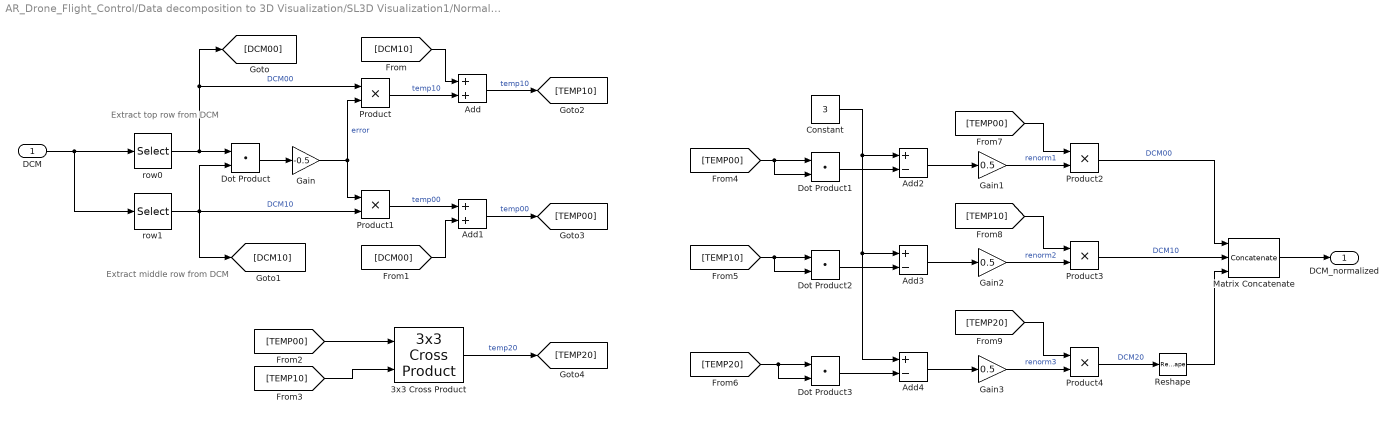
== system AR_Drone_Flight_Control/Data decomposition to 3D Visualization/SL3D Visualization1/Normalize SL3D-DCM ==
  note: Extract middle row from DCM
  note: Extract top row from DCM
  DCM : Inport  OutDataTypeStr=double  PortDimensions=[3,3]
  3x3 Cross Product : aerolibutil/3x3 Cross Product
  Add : Sum
  Add1 : Sum
  Add2 : Sum  Inputs=+-
  Add3 : Sum  Inputs=+-
  Add4 : Sum  Inputs=+-
  Constant : Constant  Value=3  OutDataTypeStr=double  SampleTime=-1
  Dot Product{,1..3} (4 alike) : DotProduct  InputSameDT=on  OutDataTypeStr=Inherit: Inherit via internal rule
  Gain : Gain  Gain=-0.5
  Gain1 : Gain  Gain=0.5  OutDataTypeStr=single
  Gain2 : Gain  Gain=0.5  OutDataTypeStr=single
  Gain3 : Gain  Gain=0.5  OutDataTypeStr=single
  Matrix Concatenate : Concatenate  NumInputs=3  Mode=Multidimensional array
  Product{,1..4} (5 alike) : Product  RndMeth=Zero
  Reshape : Reshape  OutputDimensionality=Row vector (2-D)
  row0 : Selector  NumberOfDimensions=2  IndexMode=Zero-based  InputPortWidth=3  IndexOptions=Index vector (dialog),Index vector (dialog)  Indices=0,[0:2]  OutputSizes=1,1
  row1 : Selector  NumberOfDimensions=2  IndexMode=Zero-based  InputPortWidth=3  IndexOptions=Index vector (dialog),Index vector (dialog)  Indices=1,[0:2]  OutputSizes=1,1
  DCM_normalized : Outport  OutDataTypeStr=double
  wires:
  Reshape/1 -> Matrix Concatenate/3
  Matrix Concatenate/1 -> DCM_normalized/1
  Product4/1 -> Reshape/1  "DCM20"
  Product3/1 -> Matrix Concatenate/2  "DCM10"
  Product2/1 -> Matrix Concatenate/1  "DCM00"
  [TEMP20] -> Product4/1
  [TEMP10] -> Product3/1
  [TEMP00] -> Product2/1
  Dot Product3/1 -> Add4/2
  Gain3/1 -> Product4/2  "renorm3"
  Add4/1 -> Gain3/1
  Dot Product2/1 -> Add3/2
  Gain2/1 -> Product3/2  "renorm2"
  Add3/1 -> Gain2/1
  Gain1/1 -> Product2/2  "renorm1"
  Add2/1 -> Gain1/1
  Constant/1 -> Add3/1, Add4/1, Add2/1
  Dot Product1/1 -> Add2/2
  [TEMP20] -> Dot Product3/2, Dot Product3/1
  [TEMP10] -> Dot Product2/2, Dot Product2/1
  [TEMP00] -> Dot Product1/2, Dot Product1/1
  [TEMP10] -> 3x3 Cross Product/2
  [TEMP00] -> 3x3 Cross Product/1
  3x3 Cross Product/1 -> [TEMP20]  "temp20"
  Add1/1 -> [TEMP00]  "temp00"
  Add/1 -> [TEMP10]  "temp10"
  [DCM00] -> Add1/2
  [DCM10] -> Add/1
  Product1/1 -> Add1/1  "temp00"
  Product/1 -> Add/2  "temp10"
  Gain/1 -> Product1/1, Product/2  "error"
  Dot Product/1 -> Gain/1
  row1/1 -> [DCM10], Product1/2, Dot Product/2  "DCM10"
  row0/1 -> [DCM00], Product/1, Dot Product/1  "DCM00"
  DCM/1 -> row1/1, row0/1

== system AR_Drone_Flight_Control/Data decomposition to 3D Visualization/SL3D Visualization1/SL3D DCM Output - used to adjust axes to fit wit SL3D convention ==

== system AR_Drone_Flight_Control/Flight Controller/Supervisory Flight Controller/Attitude_Control/Offset ==
  AngleIn : Inport
  Demux : Demux  Outputs=2
  Demux3 : Demux  Outputs=2
  Examine Offset At Rest : Display
  Mux1 : Mux  Inputs=2
  Offset Constants : Constant  Value=[-0.6 +0.4]*0  OutDataTypeStr=single
  Sum : Sum  Inputs=|++
  Sum1 : Sum  Inputs=|++
  AngleOut : Outport
  wires:
  Mux1/1 -> AngleOut/1
  Sum/1 -> Mux1/1
  Sum1/1 -> Mux1/2
  Demux/2 -> Sum1/1
  AngleIn/1 -> Examine Offset At Rest/1, Demux/1
  Demux3/2 -> Sum1/2
  Demux3/1 -> Sum/2
  Demux/1 -> Sum/1
  Offset Constants/1 -> Demux3/1
